simulink subsystem "Visualisation"  (R2019b)
settings: Solver=VariableStepAuto  StartTime=0.0  StopTime=10.0  RelTol=1e-3
model mask{sample_time_vis=1}
  mask prompts: sample_time_vis "sampletime"
undefined symbols (not defined in the file): ENVMT, params
settings Model: Creator=dylaneijkelhof  LastModifiedBy=dylaneijkelhof

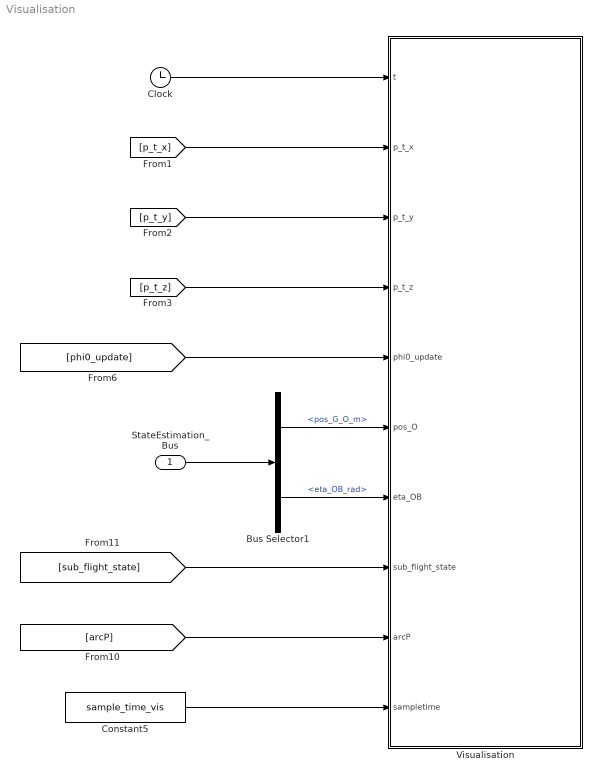
== system Visualisation ==
  StateEstimation_Bus : Inport
  Bus Selector1 : BusSelector  OutputSignals=pos_G_O_m,eta_OB_rad
  Clock : Clock
  Constant5 : Constant  Value=sample_time_vis
  Visualisation : MATLAB Function  TreatAsAtomicUnit=on
  wires:
  Clock/1 -> Visualisation/1(t)
  Bus Selector1/2 -> Visualisation/7(eta_OB)  "<eta_OB_rad>"
  [phi0_update] -> Visualisation/5(phi0_update)
  Bus Selector1/1 -> Visualisation/6(pos_O)  "<pos_G_O_m>"
  [p_t_y] -> Visualisation/3(p_t_y)
  StateEstimation_Bus/1 -> Bus Selector1/1
  [p_t_z] -> Visualisation/4(p_t_z)
  [p_t_x] -> Visualisation/2(p_t_x)
  [sub_flight_state] -> Visualisation/8(sub_flight_state)
  Constant5/1 -> Visualisation/10(sampletime)
  [arcP] -> Visualisation/9(arcP)

== matlab function Visualisation/Visualisation ==
  settings: updateMethod=DISCRETE  sampleTime=sample_time_vis
  data: t input; p_t_x input; p_t_y input; p_t_z input; phi0_update input; pos_O input; eta_OB input; params parameter; ENVMT parameter; sub_flight_state input; arcP input; sampletime input
% Copyright 2021 Delft University of Technology
%
% Licensed under the Apache License, Version 2.0 (the "License");
% you may not use this file except in compliance with the License.
% You may obtain a copy of the License at
%
%      http://www.apache.org/licenses/LICENSE-2.0
%
% Unless required by applicable law or agreed to in writing, software
% distributed under the License is distributed on an "AS IS" BASIS,
% WITHOUT WARRANTIES OR CONDITIONS OF ANY KIND, either express or implied.
% See the License for the specific language governing permissions and
% limitations under the License.

function Visualisation(t,p_t_x,p_t_y,p_t_z,phi0_update, pos_O,eta_OB,params, ENVMT, sub_flight_state, arcP, sampletime)   
    persistent handleTether
    persistent pathpoints
    persistent referencePath
    persistent Vert
    persistent handlePlane
    persistent retractionPath
    
    coder.extrinsic('plot3','patch','animatedline','addpoints');
 
    %% Figure settings
    if t==0
        figure(99)
%         addToolbarExplorationButtons(gcf)
        xlabel('x_W (m)');%, 'interpreter', 'latex')
        ylabel('y_W (m)');%, 'interpreter', 'latex')
        zlabel('z_W (m)');%, 'interpreter', 'latex')

        grid on
        box on;
        axis equal; hold on;

        view(30,21); % set the vieew angle for figure

        ax = [-500 1500];
        ay = [-1000 1000];
        az = [0 1200];
        axis([ax,ay,az]);  hold on

        X = [ax(1);ax(2);ax(2);ax(1)];
        Y = [ay(1);ay(1);ay(2);ay(2)];
        Z = [0;0;0;0];

        c = [0 1 0; % red
        0 1 0; % green
        0 1 0;
        0 1 0];
        fill3(X,Y,Z, c(:,2),'EdgeColor','none','FaceColor',c(1,:),'FaceAlpha',0.1);
    end
    
    %% Draw tether particles
    if isempty(handleTether)
 
        M_WO = [cos(ENVMT.windDirection_rad), sin(ENVMT.windDirection_rad), 0;
        sin(ENVMT.windDirection_rad), -cos(ENVMT.windDirection_rad), 0;
        0, 0, -1];
        pos_W = M_WO*[pos_O(1);pos_O(2);pos_O(3)];
        handleTether = plot3( [0;flipud(p_t_x);pos_W(1)], [0;flipud(p_t_y);pos_W(2)],[0;flipud(p_t_z);pos_W(3)],...
            '-', 'color', [0.1 0.1 0.1], 'Markersize',2, 'Linewidth', 1.2,...
            'MarkerFaceColor', [0.3 0.3 0.3]); hold on;
    end
    
    %% Draw aircraft
    if isempty(handlePlane)
        pn = pos_O(1);
        pe = pos_O(2);
        pd = pos_O(3);
        phi = eta_OB(1);
        theta = eta_OB(2);
        psi = eta_OB(3);
        
        M_WO = [cos(ENVMT.windDirection_rad), sin(ENVMT.windDirection_rad), 0;
        sin(ENVMT.windDirection_rad), -cos(ENVMT.windDirection_rad), 0;
        0, 0, -1];
        
        scale = 6;
%         [F, Vert, C] = rndread('plane_thesis_big.stl');
        Image_kite = coder.load('plane_image.mat','F','Verti','C');
        F = Image_kite.F;
        Verti = Image_kite.Verti;
        C = Image_kite.C;
        Vert = scale*Verti'; 
        V = [ cos(psi)*cos(theta) , cos(psi)*sin(phi)*sin(theta) - cos(phi)*sin(psi) , sin(phi)*sin(psi) + cos(phi)*cos(psi)*sin(theta);
            cos(theta)*sin(psi)   , cos(phi)*cos(psi) + sin(phi)*sin(psi)*sin(theta) , cos(phi)*sin(psi)*sin(theta) - cos(psi)*sin(phi);
               -sin(theta)        ,             cos(theta)*sin(phi)                  ,             cos(phi)*cos(theta)                 ]...
               * Vert;
        V = V + [pn*ones(1,size(V,2));pe*ones(1,size(V,2));pd*ones(1,size(V,2))];
        V = M_WO*V;
        col =  [ 57/255, 106/255, 177/255  ];
        handlePlane = patch('faces', F, 'vertices' ,V');
        set(handlePlane, 'facec', 'b');              % Set the face color (force it)
        set(handlePlane, 'FaceVertexCData', C);       % Set the color (from file)
        set(handlePlane, 'EdgeColor','none');
        set(handlePlane, 'FaceLighting', 'none');
        set(handlePlane, 'FaceColor', col );
    end
    
    %% Draw black thin trail behind kite
    if isempty(pathpoints)
        pathpoints = animatedline('Linestyle','-','color', [85/255, 85/255, 85/255 ], 'Linewidth', .5);
    end
    
    %% Draw red target figure of 8 (traction)
    if isempty(referencePath)
        
        Lbooth.a = params.a_booth*params.b_booth;
        Lbooth.b = params.b_booth;
        Lbooth.phi0 = phi0_update;
        
        s = 0 : 0.01 : 2*pi;
        l_tether = norm(pos_O);
        Lem.a = Lbooth.a/(l_tether); 
        Lem.b = Lbooth.b/(l_tether); 
        Lem.phi0 = Lbooth.phi0;
        long_P = Lem.b * sin(s) ./( 1+(Lem.a/Lem.b*cos(s)).^2 );
        lat_P =   Lem.a * sin(s).*cos(s) ./ ( 1+(Lem.a/Lem.b*cos(s)).^2 );
        p_P = [ cos(long_P).*cos(lat_P);sin(long_P).*cos(lat_P);sin(lat_P)]*l_tether;
        phi_p_mean = Lbooth.phi0;
        M_WP = [cos(phi_p_mean),0, -sin(phi_p_mean);0, 1, 0;  sin(phi_p_mean),0, cos(phi_p_mean)];
        p_W = M_WP * p_P;
        referencePath = plot3( p_W(1,:),p_W(2,:),p_W(3,:) , '-', 'color', [1 0.3 0.3],'Linewidth', 1.5);
    end
    
    %% Draw red retraction path (retraction)
    if isempty(retractionPath)
        retractionPath = plot3( arcP(1,:),arcP(2,:),arcP(3,:), '--', 'color', [1 0.3 0.3],'Linewidth', .5);
    end
    
    if (mod(t,sampletime)==0 && t~=0)
        %% Change each element on figure to current positions
        Lbooth.a = params.a_booth*params.b_booth;
        Lbooth.b = params.b_booth;
        Lbooth.phi0 = phi0_update;
        
        pn = pos_O(1);
        pe = pos_O(2);
        pd = pos_O(3);
        phi = eta_OB(1);
        theta = eta_OB(2);
        psi = eta_OB(3);
        
        M_WO = [cos(ENVMT.windDirection_rad), sin(ENVMT.windDirection_rad), 0;
        sin(ENVMT.windDirection_rad), -cos(ENVMT.windDirection_rad), 0;
        0, 0, -1];
        
        % Tether
        set(handleTether,'XData',[0;flipud(p_t_x);-pn], 'YData',[0;flipud(p_t_y);pe],'ZData',[0;flipud(p_t_z);-pd]);
        
        % Kite
        V = [ cos(psi)*cos(theta), cos(psi)*sin(phi)*sin(theta) - cos(phi)*sin(psi), sin(phi)*sin(psi) + cos(phi)*cos(psi)*sin(theta);
            cos(theta)*sin(psi), cos(phi)*cos(psi) + sin(phi)*sin(psi)*sin(theta), cos(phi)*sin(psi)*sin(theta) - cos(psi)*sin(phi);
            -sin(theta),                              cos(theta)*sin(phi),                              cos(phi)*cos(theta)] * Vert;
        V = V + [pn*ones(1,size(V,2));pe*ones(1,size(V,2));pd*ones(1,size(V,2))];
        V = M_WO*V;
        set(handlePlane, 'Vertices', V');
        
        % Trail
        pos_W = M_WO*[pn;pe;pd];
        addpoints(pathpoints,pos_W(1), pos_W(2),pos_W(3))
        
        % Target figure (traction)
        s = 0 : 0.01 : 2*pi;
        l_tether = norm(pos_O);
        Lem.a = Lbooth.a/(l_tether); 
        Lem.b = Lbooth.b/(l_tether); 
        Lem.phi0 = Lbooth.phi0;
        long_P = Lem.b * sin(s) ./( 1+(Lem.a/Lem.b*cos(s)).^2 );
        lat_P =   Lem.a * sin(s).*cos(s) ./ ( 1+(Lem.a/Lem.b*cos(s)).^2 );
        p_P = [ cos(long_P).*cos(lat_P);sin(long_P).*cos(lat_P);sin(lat_P)]*l_tether;
        phi_p_mean = Lbooth.phi0;
        M_WP = [cos(phi_p_mean),0, -sin(phi_p_mean);0, 1, 0;  sin(phi_p_mean),0, cos(phi_p_mean)];
        p_W = M_WP * p_P;
        set(referencePath,'XData',p_W(1,:),'YData',p_W(2,:),'ZData',p_W(3,:));
        
        % Target path (retraction)
        if sub_flight_state >= 6
            set(retractionPath,'XData',arcP(1,:),'YData',arcP(2,:),'ZData',arcP(3,:));
        else
            set(retractionPath,'XData',zeros(1,size(arcP,2)),'YData',zeros(1,size(arcP,2)),'ZData',zeros(1,size(arcP,2)));
        end
    end
